simulink model "implementing_equations"  (R2024a)
settings: Solver=VariableStepAuto  StartTime=0.0  StopTime=10.0  RelTol=1e-3
values from neighbouring files (symbols this model uses):
  A = 3    [implementing_equations_script.m]
  F = 2    [implementing_equations_script.m]
  Ti = 0.5    [implementing_equations_script.m]
settings Model: Creator=robin  LastModifiedBy=robin

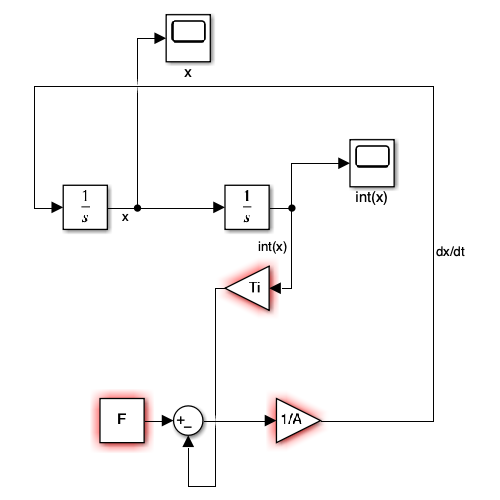
[thumbnail: Simulink's stored preview of the top-level diagram]
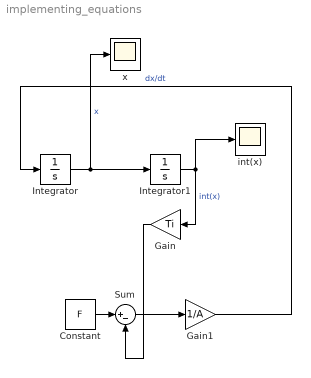
== system implementing_equations ==
  Constant : Constant  Value=F
  Gain : Gain  Gain=Ti
  Gain1 : Gain  Gain=1/A
  Integrator : Integrator
  Integrator1 : Integrator
  Sum : Sum  Inputs=|+-
  int(x) : Scope
  x : Scope
  wires:
  Integrator/1 -> Integrator1/1, x/1  "x"
  Constant/1 -> Sum/1
  Integrator1/1 -> Gain/1, int(x)/1  "int(x)"
  Gain/1 -> Sum/2
  Sum/1 -> Gain1/1
  Gain1/1 -> Integrator/1  "dx/dt"
